simulink model "calc_c1_coefficients_sim"  (R2020b)
settings: Solver=FixedStepDiscrete  StartTime=0.0  StopTime=stopTime  RelTol=1e-3
InitFcn:
  | initCallback
StopFcn:
  | stopCallback
undefined symbols (not defined in the file or in its folder): mp
settings Model: Creator=Ross  LastModifiedBy=conno
settings DataIOCC: ReturnWorkspaceOutputs=off
settings OptimizationCC: BlockReduction=off  ConditionallyExecuteInputs=off  DefaultParameterBehavior=Inlined
settings DebuggingCC: ReadBeforeWriteMsg=DisableAll  WriteAfterWriteMsg=DisableAll  WriteAfterReadMsg=DisableAll  AlgebraicLoopMsg=error  MultiTaskDSMMsg=none  SingleTaskRateTransMsg=error  PregeneratedLibrarySubsystemCodeDiagnostic=none  ArithmeticOperatorsInVariantConditions=warning
settings HardwareCC: ProdBitPerPointer=32  ProdBitPerSizeT=32  ProdBitPerPtrDiffT=32  ProdLargestAtomicFloat=None  ProdIntDivRoundTo=Undefined  ProdEndianess=Unspecified  ProdWordSize=32  ProdHWDeviceType=ASIC/FPGA->ASIC/FPGA  TargetBitPerPointer=64  TargetBitPerSizeT=64  TargetBitPerPtrDiffT=64  TargetLongLongMode=on  TargetIntDivRoundTo=Zero  TargetEndianess=LittleEndian  TargetWordSize=64  TargetHWDeviceType=Custom Processor->MATLAB Host Computer  ProdEqTarget=off
settings ModelReferenceCC: UpdateModelReferenceTargets=IfOutOfDate
settings SFSimCC: SFSimEcho=off  SimUseLocalCustomCode=off  CustomCodeUndefinedFunction=UseInterfaceOnly
settings RTWCC: RTWUseLocalCustomCode=off

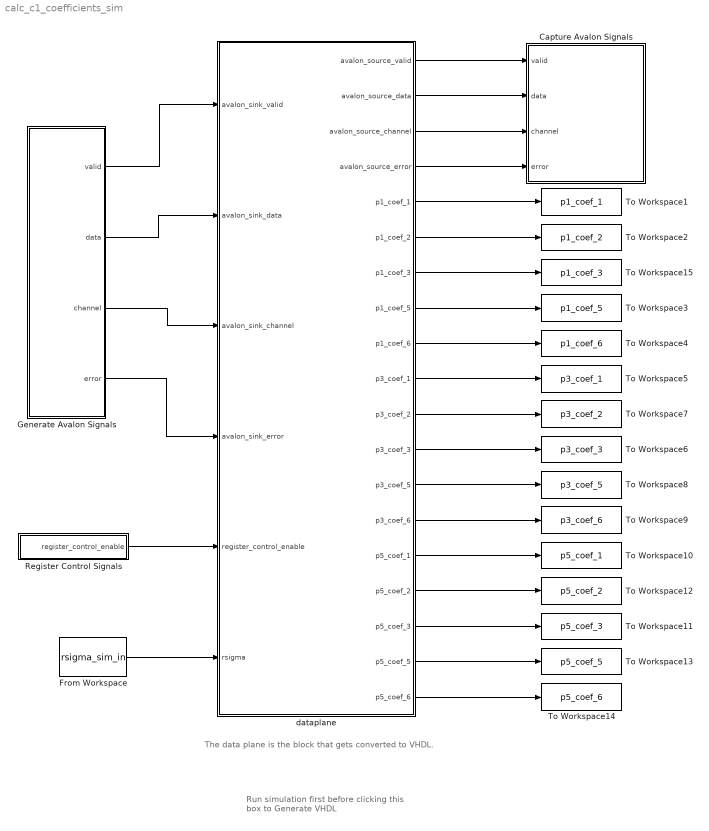
== system calc_c1_coefficients_sim ==
  note: The data plane is the block that gets converted to VHDL.
  note: Run simulation first
      | before clicking this box to
      | Generate VHDL
  Capture Avalon Signals : Subsystem
  From Workspace : FromWorkspace  VariableName=rsigma_sim_in  SampleTime=-1
  Generate Avalon Signals : Subsystem
  Register Control Signals : Subsystem
  To Workspace1 : ToWorkspace  VariableName=p1_coef_1  SampleTime=-1
  To Workspace10 : ToWorkspace  VariableName=p5_coef_1  SampleTime=-1
  To Workspace11 : ToWorkspace  VariableName=p5_coef_3  SampleTime=-1
  To Workspace12 : ToWorkspace  VariableName=p5_coef_2  SampleTime=-1
  To Workspace13 : ToWorkspace  VariableName=p5_coef_5  SampleTime=-1
  To Workspace14 : ToWorkspace  VariableName=p5_coef_6  SampleTime=-1
  To Workspace15 : ToWorkspace  VariableName=p1_coef_3  SampleTime=-1
  To Workspace2 : ToWorkspace  VariableName=p1_coef_2  SampleTime=-1
  To Workspace3 : ToWorkspace  VariableName=p1_coef_5  SampleTime=-1
  To Workspace4 : ToWorkspace  VariableName=p1_coef_6  SampleTime=-1
  To Workspace5 : ToWorkspace  VariableName=p3_coef_1  SampleTime=-1
  To Workspace6 : ToWorkspace  VariableName=p3_coef_3  SampleTime=-1
  To Workspace7 : ToWorkspace  VariableName=p3_coef_2  SampleTime=-1
  To Workspace8 : ToWorkspace  VariableName=p3_coef_5  SampleTime=-1
  To Workspace9 : ToWorkspace  VariableName=p3_coef_6  SampleTime=-1
  dataplane : Subsystem  TreatAsAtomicUnit=on
  wires:
  Generate Avalon Signals/2(data) -> dataplane/2(avalon_sink_data)
  Generate Avalon Signals/1(valid) -> dataplane/1(avalon_sink_valid)
  Generate Avalon Signals/3(channel) -> dataplane/3(avalon_sink_channel)
  Generate Avalon Signals/4(error) -> dataplane/4(avalon_sink_error)
  dataplane/2(avalon_source_data) -> Capture Avalon Signals/2(data)
  dataplane/1(avalon_source_valid) -> Capture Avalon Signals/1(valid)
  dataplane/3(avalon_source_channel) -> Capture Avalon Signals/3(channel)
  dataplane/4(avalon_source_error) -> Capture Avalon Signals/4(error)
  Register Control Signals/1(register_control_enable) -> dataplane/5(register_control_enable)
  From Workspace/1 -> dataplane/6(rsigma)
  dataplane/5(p1_coef_1) -> To Workspace1/1
  dataplane/6(p1_coef_2) -> To Workspace2/1
  dataplane/7(p1_coef_3) -> To Workspace15/1
  dataplane/8(p1_coef_5) -> To Workspace3/1
  dataplane/9(p1_coef_6) -> To Workspace4/1
  dataplane/10(p3_coef_1) -> To Workspace5/1
  dataplane/11(p3_coef_2) -> To Workspace7/1
  dataplane/12(p3_coef_3) -> To Workspace6/1
  dataplane/13(p3_coef_5) -> To Workspace8/1
  dataplane/14(p3_coef_6) -> To Workspace9/1
  dataplane/15(p5_coef_1) -> To Workspace10/1
  dataplane/16(p5_coef_2) -> To Workspace12/1
  dataplane/17(p5_coef_3) -> To Workspace11/1
  dataplane/18(p5_coef_5) -> To Workspace13/1
  dataplane/19(p5_coef_6) -> To Workspace14/1

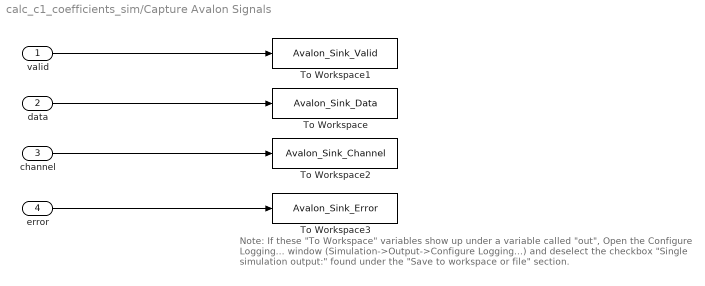
== system calc_c1_coefficients_sim/Capture Avalon Signals ==
  note: Note:  If these "To Workspace" variables show up under a variable called "out",
      | Open the Configure Logging... window (Simulation->Output->Configure Logging...)
      | and deselect the checkbox "Single simulation output:" found under the "Save to workspace or file" section.
  valid : Inport
  data : Inport  Port=2
  channel : Inport  Port=3
  error : Inport  Port=4
  To Workspace : ToWorkspace  VariableName=Avalon_Sink_Data  SaveFormat=Timeseries  SampleTime=-1
  To Workspace1 : ToWorkspace  VariableName=Avalon_Sink_Valid  SaveFormat=Timeseries  SampleTime=-1
  To Workspace2 : ToWorkspace  VariableName=Avalon_Sink_Channel  SaveFormat=Timeseries  SampleTime=-1
  To Workspace3 : ToWorkspace  VariableName=Avalon_Sink_Error  SaveFormat=Timeseries  SampleTime=-1
  wires:
  data/1 -> To Workspace/1
  valid/1 -> To Workspace1/1
  error/1 -> To Workspace3/1
  channel/1 -> To Workspace2/1

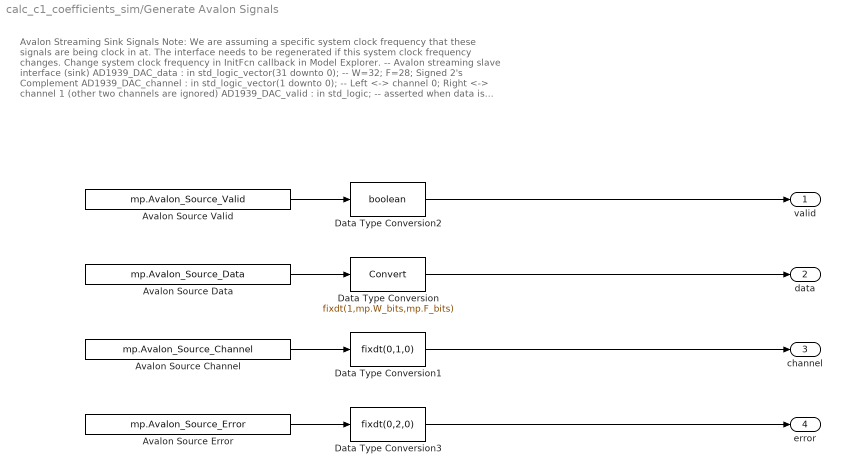
== system calc_c1_coefficients_sim/Generate Avalon Signals ==
  note: Avalon Streaming Sink Signals
      | Note: We are assuming a specific system clock frequency that these signals are being clock in at.
      | The interface needs to be regenerated if this system clock frequency changes. Change system clock frequency in InitFcn callback in Model Explorer.
      |
      | -- Avalon streaming slave interface (sink)
      | AD1939_DAC_data : in std_logic_vector(31 downto 0); -- W=32; F=28; Signed 2's Complement
      | AD1939_DAC_channel : in std_logic_vector(1 downto 0); -- Left <-> channel 0; Right <-> channel 1 (other two channels are ignored)
      | AD1939_DAC_valid : in std_logic; -- asserted when data is valid
      | AD1939_DAC_error : in std_logic_vector(1 downto 0) -- error channel is ignored, assumed to be error free at this point
      |
      | For more information on the data-channel-valid protocol, s ee chapter 5 in Intel's Avalon Interfaced Specification (p. 40) at https://www.intel.com/content/dam/www/programmable/us/en/pdfs/literature/manual/mnl_avalon_spec.pdf
  Avalon Source Channel : FromWorkspace  VariableName=mp.Avalon_Source_Channel  OutDataTypeStr=double  SampleTime=mp.Ts_sim
  "Avalon Source Data " : FromWorkspace  VariableName=mp.Avalon_Source_Data  OutDataTypeStr=double  SampleTime=mp.Ts_sim
  Avalon Source Error : FromWorkspace  VariableName=mp.Avalon_Source_Error  OutDataTypeStr=double  SampleTime=mp.Ts_sim
  Avalon Source Valid : FromWorkspace  VariableName=mp.Avalon_Source_Valid  OutDataTypeStr=double  SampleTime=mp.Ts_sim
  Data Type Conversion : DataTypeConversion  OutDataTypeStr=fixdt(1,mp.W_bits,mp.F_bits)
  Data Type Conversion1 : DataTypeConversion  OutDataTypeStr=fixdt(0,1,0)
  Data Type Conversion2 : DataTypeConversion  OutDataTypeStr=boolean
  Data Type Conversion3 : DataTypeConversion  OutDataTypeStr=fixdt(0,2,0)
  valid : Outport  VectorParamsAs1DForOutWhenUnconnected=off
  data : Outport  Port=2  VectorParamsAs1DForOutWhenUnconnected=off
  channel : Outport  Port=3  VectorParamsAs1DForOutWhenUnconnected=off
  error : Outport  Port=4  VectorParamsAs1DForOutWhenUnconnected=off
  wires:
  Data Type Conversion1/1 -> channel/1
  Data Type Conversion2/1 -> valid/1
  Avalon Source Error/1 -> Data Type Conversion3/1
  Data Type Conversion/1 -> data/1
  Avalon Source Valid/1 -> Data Type Conversion2/1
  Data Type Conversion3/1 -> error/1
  Avalon Source Channel/1 -> Data Type Conversion1/1
  "Avalon Source Data "/1 -> Data Type Conversion/1

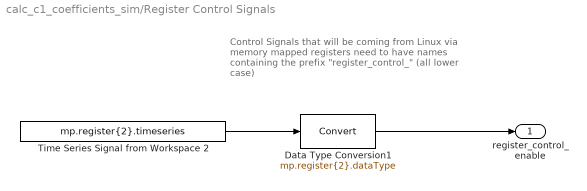
== system calc_c1_coefficients_sim/Register Control Signals ==
  note: Control Signals that will be coming from Linux via
      | memory mapped registers need to have names
      | containing the prefix "register_control_"
      | (all lower case)
  Data Type Conversion1 : DataTypeConversion  OutDataTypeStr=mp.register{2}.dataType
  Time Series Signal from Workspace 2 : FromWorkspace  VariableName=mp.register{2}.timeseries  OutDataTypeStr=double  SampleTime=mp.Ts_sim
  register_control_enable : Outport  VectorParamsAs1DForOutWhenUnconnected=off
  wires:
  Data Type Conversion1/1 -> register_control_enable/1
  Time Series Signal from Workspace 2/1 -> Data Type Conversion1/1

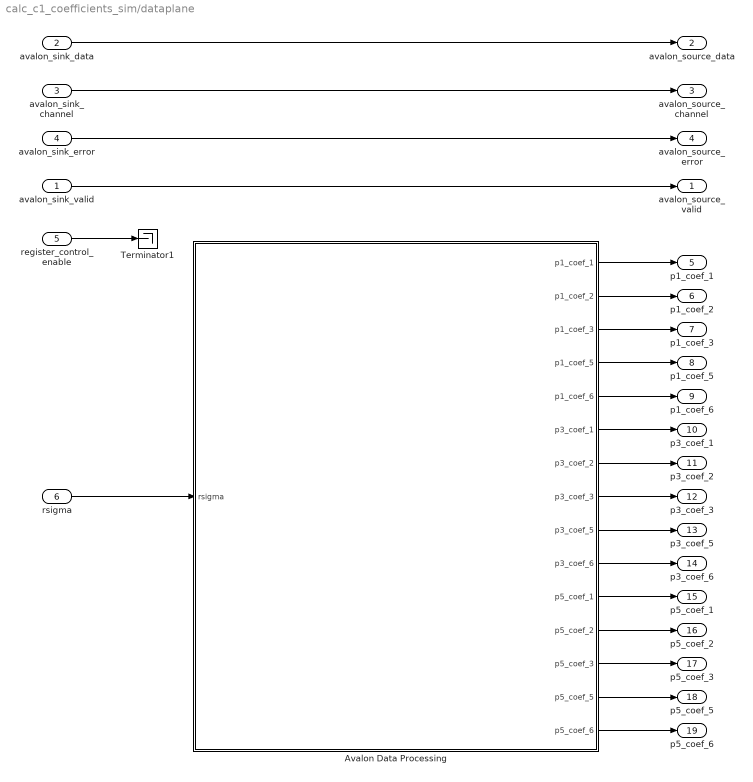
== system calc_c1_coefficients_sim/dataplane ==
  avalon_sink_valid : Inport
  avalon_sink_data : Inport  Port=2
  avalon_sink_channel : Inport  Port=3
  avalon_sink_error : Inport  Port=4
  register_control_enable : Inport  Port=5
  rsigma : Inport  Port=6
  Avalon Data Processing : Subsystem  TreatAsAtomicUnit=on
  Terminator1 : Terminator
  avalon_source_valid : Outport  VectorParamsAs1DForOutWhenUnconnected=off
  avalon_source_data : Outport  Port=2  VectorParamsAs1DForOutWhenUnconnected=off
  avalon_source_channel : Outport  Port=3  VectorParamsAs1DForOutWhenUnconnected=off
  avalon_source_error : Outport  Port=4  VectorParamsAs1DForOutWhenUnconnected=off
  p1_coef_1 : Outport  Port=5
  p1_coef_2 : Outport  Port=6
  p1_coef_3 : Outport  Port=7
  p1_coef_5 : Outport  Port=8
  p1_coef_6 : Outport  Port=9
  p3_coef_1 : Outport  Port=10
  p3_coef_2 : Outport  Port=11
  p3_coef_3 : Outport  Port=12
  p3_coef_5 : Outport  Port=13
  p3_coef_6 : Outport  Port=14
  p5_coef_1 : Outport  Port=15
  p5_coef_2 : Outport  Port=16
  p5_coef_3 : Outport  Port=17
  p5_coef_5 : Outport  Port=18
  p5_coef_6 : Outport  Port=19
  wires:
  avalon_sink_error/1 -> avalon_source_error/1
  avalon_sink_valid/1 -> avalon_source_valid/1
  avalon_sink_channel/1 -> avalon_source_channel/1
  register_control_enable/1 -> Terminator1/1
  rsigma/1 -> Avalon Data Processing/1(rsigma)
  avalon_sink_data/1 -> avalon_source_data/1
  Avalon Data Processing/15(p5_coef_6) -> p5_coef_6/1
  Avalon Data Processing/14(p5_coef_5) -> p5_coef_5/1
  Avalon Data Processing/13(p5_coef_3) -> p5_coef_3/1
  Avalon Data Processing/12(p5_coef_2) -> p5_coef_2/1
  Avalon Data Processing/11(p5_coef_1) -> p5_coef_1/1
  Avalon Data Processing/10(p3_coef_6) -> p3_coef_6/1
  Avalon Data Processing/9(p3_coef_5) -> p3_coef_5/1
  Avalon Data Processing/8(p3_coef_3) -> p3_coef_3/1
  Avalon Data Processing/7(p3_coef_2) -> p3_coef_2/1
  Avalon Data Processing/6(p3_coef_1) -> p3_coef_1/1
  Avalon Data Processing/5(p1_coef_6) -> p1_coef_6/1
  Avalon Data Processing/4(p1_coef_5) -> p1_coef_5/1
  Avalon Data Processing/3(p1_coef_3) -> p1_coef_3/1
  Avalon Data Processing/2(p1_coef_2) -> p1_coef_2/1
  Avalon Data Processing/1(p1_coef_1) -> p1_coef_1/1

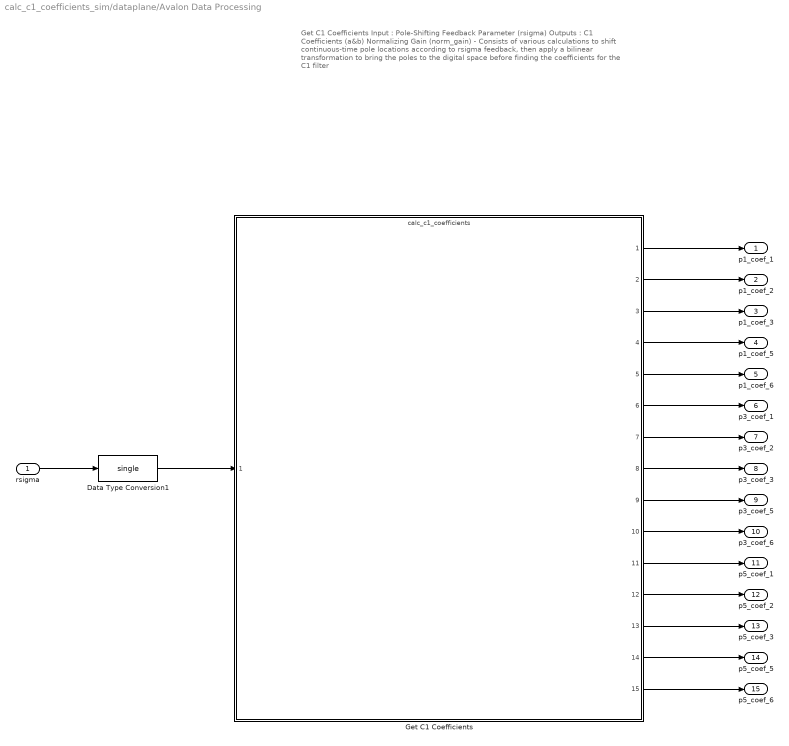
== system calc_c1_coefficients_sim/dataplane/Avalon Data Processing ==
  note: Get C1 Coefficients
      |
      | Input : Pole-Shifting Feedback Parameter (rsigma)
      |
      | Outputs : C1 Coefficients (a&b)
      | Normalizing Gain (norm_gain)
      |
      | - Consists of various calculations to shift continuous-time pole locations according to rsigma feedback, then apply a bilinear transformation to bring the poles to the digital space before finding the coefficients for the C1 filter
  rsigma : Inport
  Data Type Conversion1 : DataTypeConversion  OutDataTypeStr=single  RndMeth=Nearest
  Get C1 Coefficients : ModelReference  ModelNameDialog=calc_c1_coefficients  SimulationMode=Normal  ModelReferenceVersion=1.151
  p1_coef_1 : Outport
  p1_coef_2 : Outport  Port=2
  p1_coef_3 : Outport  Port=3
  p1_coef_5 : Outport  Port=4
  p1_coef_6 : Outport  Port=5
  p3_coef_1 : Outport  Port=6
  p3_coef_2 : Outport  Port=7
  p3_coef_3 : Outport  Port=8
  p3_coef_5 : Outport  Port=9
  p3_coef_6 : Outport  Port=10
  p5_coef_1 : Outport  Port=11
  p5_coef_2 : Outport  Port=12
  p5_coef_3 : Outport  Port=13
  p5_coef_5 : Outport  Port=14
  p5_coef_6 : Outport  Port=15
  wires:
  rsigma/1 -> Data Type Conversion1/1
  Data Type Conversion1/1 -> Get C1 Coefficients/1
  Get C1 Coefficients/2 -> p1_coef_2/1
  Get C1 Coefficients/3 -> p1_coef_3/1
  Get C1 Coefficients/4 -> p1_coef_5/1
  Get C1 Coefficients/5 -> p1_coef_6/1
  Get C1 Coefficients/1 -> p1_coef_1/1
  Get C1 Coefficients/10 -> p3_coef_6/1
  Get C1 Coefficients/9 -> p3_coef_5/1
  Get C1 Coefficients/8 -> p3_coef_3/1
  Get C1 Coefficients/7 -> p3_coef_2/1
  Get C1 Coefficients/6 -> p3_coef_1/1
  Get C1 Coefficients/15 -> p5_coef_6/1
  Get C1 Coefficients/14 -> p5_coef_5/1
  Get C1 Coefficients/13 -> p5_coef_3/1
  Get C1 Coefficients/12 -> p5_coef_2/1
  Get C1 Coefficients/11 -> p5_coef_1/1
